simulink model "ModeInputHandle"  (R2018b)
settings: Solver=FixedStepDiscrete  StartTime=0.0  StopTime=10.0  FixedStep=0.01  RelTol=1e-3
undefined symbols (not defined in the file or in its folder): c, CmprtMdHMIReqExt2Tp1, CmprtMdHMIReqExtTp1, CmprtMdHMIReqTp1, d, e, EZESwReq1, f, g, IfVeSMSeStNumConfig, j, KeSMSuButtonLongPressedThrshldTm_Val, KeSMSuFoldType_Val, KeSMSwSeatSMSSeatMdTrigGapTimer_Val, KeSMSwSeatTrigWaitTimer_Val, KeSMSwSRSActiveValidTm_Val, LckUlckActvtFunc1, LstLckFunc1, LugSelectSw1, MdReqTp1, PowerMode1, SeatOccupiedSts1, SRSMode1, StPassCmprtMdCtrl_Md10_VCUConfig_Val, StPassCmprtMdCtrl_Md11_VCUConfig_Val, StPassCmprtMdCtrl_Md12_VCUConfig_Val, StPassCmprtMdCtrl_Md13_VCUConfig_Val, StPassCmprtMdCtrl_Md1_VCUConfig_Val, StPassCmprtMdCtrl_Md27_VCUConfig_Val, StPassCmprtMdCtrl_Md28_VCUConfig_Val, StPassCmprtMdCtrl_Md29_VCUConfig_Val, StPassCmprtMdCtrl_Md2_VCUConfig_Val, StPassCmprtMdCtrl_Md30_VCUConfig_Val, StPassCmprtMdCtrl_Md31_VCUConfig_Val, StPassCmprtMdCtrl_Md32_VCUConfig_Val, StPassCmprtMdCtrl_Md3_VCUConfig_Val, StPassCmprtMdCtrl_Md53_VCUConfig_Val, StPassCmprtMdCtrl_Md56_VCUConfig_Val, StPassCmprtMdCtrl_Md57_VCUConfig_Val, StPassCmprtMdCtrl_Md58_VCUConfig_Val, StPassCmprtMdCtrl_Md61_VCUConfig_Val, StPassCmprtMdCtrl_Md62_VCUConfig_Val, StPassCmprtMdCtrl_Md8_VCUConfig_Val, StPassCmprtMdCtrl_Md9_VCUConfig_Val, StSrv_StMd10_Config_Val, StSrv_StMd11_Config_Val, StSrv_StMd12_Config_Val, StSrv_StMd13_Config_Val, StSrv_StMd1_Config_Val, StSrv_StMd27_Config_Val, StSrv_StMd28_Config_Val, StSrv_StMd29_Config_Val, StSrv_StMd2_Config_Val, StSrv_StMd30_Config_Val, StSrv_StMd31_Config_Val, StSrv_StMd32_Config_Val, StSrv_StMd3_Config_Val, StSrv_StMd8_Config_Val, StSrv_StMd9_Config_Val, VehMovState1
libraries: MSMLib x91
(part 6 of 9)

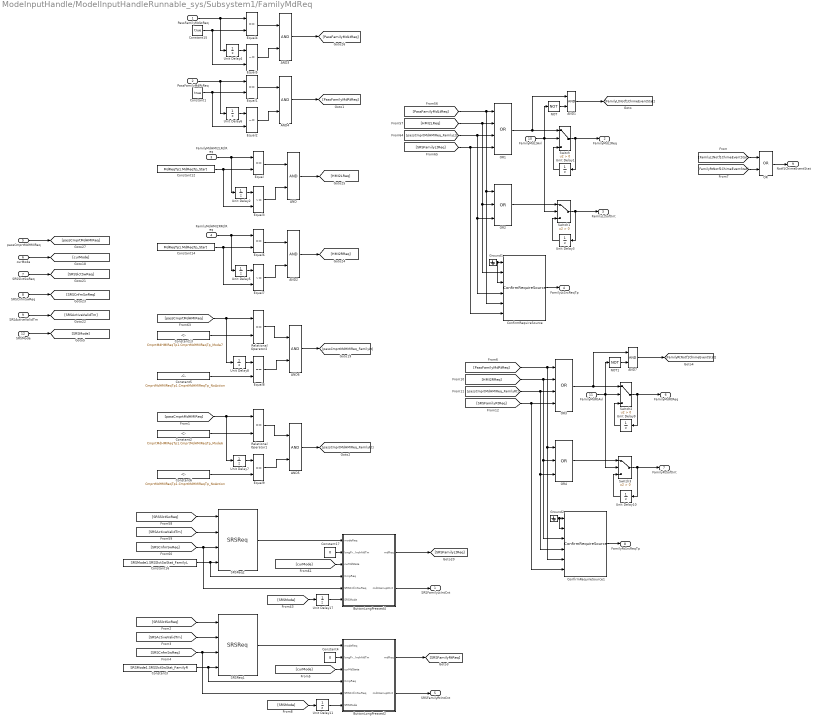
== system ModeInputHandle/ModelInputHandleRunnable_sys/Subsystem1/FamilyMdReq ==
  PassFamilyMdLtReq : Inport
  PassFamilyMdRtReq : Inport  Port=2
  FamilyMdHMI2LRclReq : Inport  Port=3
  FamilyMdHMI2RRclReq : Inport  Port=4
  passCmprtMdHMIReq : Inport  Port=5
  curMode : Inport  Port=6
  SRSSlctSwReq : Inport  Port=7
  SRSCnfmSwReq : Inport  Port=8
  SRSActiveValidTm : Inport  Port=9
  FamilyMdLtAvl : Inport  Port=10
  FamilyMdRtAvl : Inport  Port=11
  SRSMode : Inport  Port=12
  AND{,1..7} (8 alike) : Logic  AllPortsSameDT=off  OutDataTypeStr=boolean
  ButtonLongPressed2 : Subsystem  AncestorBlock=MSMLib/ButtonLongPressed
  ButtonLongPressed4 : Subsystem  AncestorBlock=MSMLib/ButtonLongPressed
  ConfirmRequireSource : MSMLib/ConfirmRequireSource  SystemSampleTime=-1
  ConfirmRequireSource1 : MSMLib/ConfirmRequireSource  SystemSampleTime=-1
  Constant1 : Constant  Value=true  OutDataTypeStr=boolean
  Constant12 : Constant  Value=MdReqTp1.MdReqTp_Start
  Constant13 : Constant  Value=CmprtMdHMIReqTp1.CmprtMdHMIReqTp_Mode7  OutDataTypeStr=Enum:CmprtMdHMIReqTp1
  Constant14 : Constant  Value=MdReqTp1.MdReqTp_Start
  Constant15 : Constant  Value=true  OutDataTypeStr=boolean
  Constant16 : Constant  Value=SRSMode1.SRSSlctSwStat_FamilyL  OutDataTypeStr=Enum:SRSMode1
  Constant17 : Constant  Value=0  OutDataTypeStr=uint8
  Constant2 : Constant  Value=CmprtMdHMIReqTp1.CmprtMdHMIReqTp_Mode6  OutDataTypeStr=Enum:CmprtMdHMIReqTp1
  Constant3 : Constant  Value=SRSMode1.SRSSlctSwStat_FamilyR  OutDataTypeStr=Enum:SRSMode1
  Constant4 : Constant  Value=0  OutDataTypeStr=uint8
  Constant5 : Constant  Value=CmprtMdHMIReqTp1.CmprtMdHMIReqTp_NoAction  OutDataTypeStr=Enum:CmprtMdHMIReqTp1
  Constant6 : Constant  Value=CmprtMdHMIReqTp1.CmprtMdHMIReqTp_NoAction  OutDataTypeStr=Enum:CmprtMdHMIReqTp1
  Equal{,1,4,6,8..9} (6 alike) : RelationalOperator  Operator===  OutDataTypeStr=boolean  RndMeth=Simplest
  Equal{2..3,5,7} (4 alike) : RelationalOperator  Operator=~=  OutDataTypeStr=boolean  RndMeth=Simplest
  Ground1 : Ground
  Ground2 : Ground
  NOT : Logic  Operator=NOT  AllPortsSameDT=off  OutDataTypeStr=boolean
  NOT1 : Logic  Operator=NOT  AllPortsSameDT=off  OutDataTypeStr=boolean
  OR : Logic  Operator=OR  AllPortsSameDT=off  OutDataTypeStr=boolean
  OR1 : Logic  Operator=OR  Inputs=4  AllPortsSameDT=off  OutDataTypeStr=boolean
  OR2 : Logic  Operator=OR  Inputs=3  AllPortsSameDT=off  OutDataTypeStr=boolean
  OR3 : Logic  Operator=OR  Inputs=4  AllPortsSameDT=off  OutDataTypeStr=boolean
  OR4 : Logic  Operator=OR  Inputs=3  AllPortsSameDT=off  OutDataTypeStr=boolean
  Relational Operator1 : RelationalOperator  Operator===  OutDataTypeStr=boolean  RndMeth=Simplest
  Relational Operator2 : RelationalOperator  Operator===  OutDataTypeStr=boolean  RndMeth=Simplest
  SRSReq1 : MSMLib/SRSReq  SystemSampleTime=-1
  SRSReq2 : MSMLib/SRSReq  SystemSampleTime=-1
  Switch{,1..3} (4 alike) : Switch  Criteria=u2 > Threshold
  Unit Delay{1,3..4,6,9..10} (6 alike) : UnitDelay  SampleTime=-1
  Unit Delay11 : UnitDelay  InitialCondition=d  SampleTime=-1
  Unit Delay17 : UnitDelay  InitialCondition=d  SampleTime=-1
  Unit Delay2 : UnitDelay  InitialCondition=e  SampleTime=-1
  Unit Delay5 : UnitDelay  InitialCondition=e  SampleTime=-1
  Unit Delay7 : UnitDelay  InitialCondition=c  SampleTime=-1
  Unit Delay8 : UnitDelay  InitialCondition=c  SampleTime=-1
  SRSFamilyLtIntCnt : Outport
  FamilyMdLtReq : Outport  Port=2
  FamilyLtSoftInt : Outport  Port=3
  FamilyLtSrcReqTp : Outport  Port=4
  SRSFamilyRtIntCnt : Outport  Port=5
  FamilyMdRtReq : Outport  Port=6
  FamilyRtSoftInt : Outport  Port=7
  FamilyRtSrcReqTp : Outport  Port=8
  Notf1ChimeEventStat : Outport  Port=9
  wires:
  FamilyMdLtAvl/1 -> Switch1/2, NOT/1, Switch/2
  [SRSActiveValidTm] -> SRSReq2/2
  Unit Delay2/1 -> Equal3/1
  FamilyMdHMI2LRclReq/1 -> Unit Delay2/1, Equal/1
  Constant14/1 -> Equal7/2, Equal6/2
  Equal5/1 -> AND3/2
  Constant16/1 -> ButtonLongPressed4/4(CmpReq), SRSReq2/4
  Equal6/1 -> AND2/1
  Equal/1 -> AND/1
  AND3/1 -> [PassFamilyMdLtReq]
  PassFamilyMdLtReq/1 -> Unit Delay4/1, Equal4/1
  [SRSCnfmSwReq] -> ButtonLongPressed4/5(SRSCnfmSwReq), SRSReq2/3
  Constant17/1 -> ButtonLongPressed4/2(longPressThrshhldTm)
  [PassFamilyMdLtReq] -> ConfirmRequireSource/5, OR2/1, OR1/1
  Equal3/1 -> AND/2
  SRSSlctSwReq/1 -> [SRSSlctSwReq]
  OR1/1 -> AND1/1, Switch/1
  FamilyMdHMI2RRclReq/1 -> Unit Delay5/1, Equal6/1
  Constant13/1 -> Relational Operator2/2
  [curMode] -> ButtonLongPressed4/3(curMdState)
  Equal4/1 -> AND3/1
  Constant12/1 -> Equal3/2, Equal/2
  curMode/1 -> [curMode]
  [passCmprtMdHMIReq] -> Unit Delay8/1, Relational Operator2/1
  AND1/1 -> [FamilyLtNotf1ChimeEventStat]
  SRSActiveValidTm/1 -> [SRSActiveValidTm]
  OR2/1 -> Switch1/1
  Equal7/1 -> AND2/2
  Switch/1 -> FamilyMdLtReq/1, Unit Delay1/1
  Constant15/1 -> Equal4/2, Equal5/2
  Unit Delay5/1 -> Equal7/1
  ButtonLongPressed4/1(mdReq) -> [SRSFamilyLtReq]
  Unit Delay1/1 -> Switch/3
  AND6/1 -> [passCmprtMdHMIReq_FamilyLt]
  ConfirmRequireSource/1 -> FamilyLtSrcReqTp/1
  SRSCnfmSwReq/1 -> [SRSCnfmSwReq]
  Switch1/1 -> FamilyLtSoftInt/1, Unit Delay3/1
  Ground1/1 -> ConfirmRequireSource/3, ConfirmRequireSource/1
  Unit Delay4/1 -> Equal5/1
  NOT/1 -> AND1/2
  ButtonLongPressed4/2(mdInterruptCnt) -> SRSFamilyLtIntCnt/1
  AND2/1 -> [HMI2RReq]
  Unit Delay8/1 -> Equal8/1
  [SRSSlctSwReq] -> SRSReq2/1
  Equal8/1 -> AND6/2
  AND/1 -> [HMI2LReq]
  SRSReq2/1 -> ButtonLongPressed4/1(modeReq)
  passCmprtMdHMIReq/1 -> [passCmprtMdHMIReq]
  Unit Delay3/1 -> Switch1/3
  Relational Operator2/1 -> AND6/1
  Unit Delay6/1 -> Equal2/1
  Equal1/1 -> AND4/1
  Equal2/1 -> AND4/2
  PassFamilyMdRtReq/1 -> Unit Delay6/1, Equal1/1
  Constant1/1 -> Equal1/2, Equal2/2
  AND4/1 -> [PassFamilyMdRtReq]
  [passCmprtMdHMIReq] -> Unit Delay7/1, Relational Operator1/1
  Relational Operator1/1 -> AND5/1
  Equal9/1 -> AND5/2
  Constant2/1 -> Relational Operator1/2
  Unit Delay7/1 -> Equal9/1
  AND5/1 -> [passCmprtMdHMIReq_FamilyRt]
  SRSReq1/1 -> ButtonLongPressed2/1(modeReq)
  [SRSSlctSwReq] -> SRSReq1/1
  [curMode] -> ButtonLongPressed2/3(curMdState)
  Constant4/1 -> ButtonLongPressed2/2(longPressThrshhldTm)
  [SRSActiveValidTm] -> SRSReq1/2
  Constant3/1 -> ButtonLongPressed2/4(CmpReq), SRSReq1/4
  ButtonLongPressed2/1(mdReq) -> [SRSFamilyRtReq]
  [SRSCnfmSwReq] -> ButtonLongPressed2/5(SRSCnfmSwReq), SRSReq1/3
  ButtonLongPressed2/2(mdInterruptCnt) -> SRSFamilyRtIntCnt/1
  [HMI2LReq] -> ConfirmRequireSource/2, OR2/2, OR1/2
  [passCmprtMdHMIReq_FamilyLt] -> ConfirmRequireSource/4, OR2/3, OR1/3
  [SRSFamilyLtReq] -> ConfirmRequireSource/6, OR1/4
  Switch3/1 -> FamilyRtSoftInt/1, Unit Delay10/1
  Unit Delay10/1 -> Switch3/3
  NOT1/1 -> AND7/2
  OR3/1 -> AND7/1, Switch2/1
  [PassFamilyMdRtReq] -> ConfirmRequireSource1/5, OR4/1, OR3/1
  [passCmprtMdHMIReq_FamilyRt] -> ConfirmRequireSource1/4, OR4/3, OR3/3
  Ground2/1 -> ConfirmRequireSource1/2, ConfirmRequireSource1/1
  ConfirmRequireSource1/1 -> FamilyRtSrcReqTp/1
  [SRSFamilyRtReq] -> ConfirmRequireSource1/6, OR3/4
  Switch2/1 -> FamilyMdRtReq/1, Unit Delay9/1
  OR4/1 -> Switch3/1
  FamilyMdRtAvl/1 -> Switch3/2, NOT1/1, Switch2/2
  Unit Delay9/1 -> Switch2/3
  AND7/1 -> [FamilyRtNotf1ChimeEventStat]
  [HMI2RReq] -> ConfirmRequireSource1/3, OR4/2, OR3/2
  [FamilyLtNotf1ChimeEventStat] -> OR/1
  [FamilyRtNotf1ChimeEventStat] -> OR/2
  OR/1 -> Notf1ChimeEventStat/1
  Unit Delay17/1 -> ButtonLongPressed4/6(SRSMode)
  [SRSMode] -> Unit Delay17/1
  Unit Delay11/1 -> ButtonLongPressed2/6(SRSMode)
  [SRSMode] -> Unit Delay11/1
  SRSMode/1 -> [SRSMode]
  Constant5/1 -> Equal8/2
  Constant6/1 -> Equal9/2

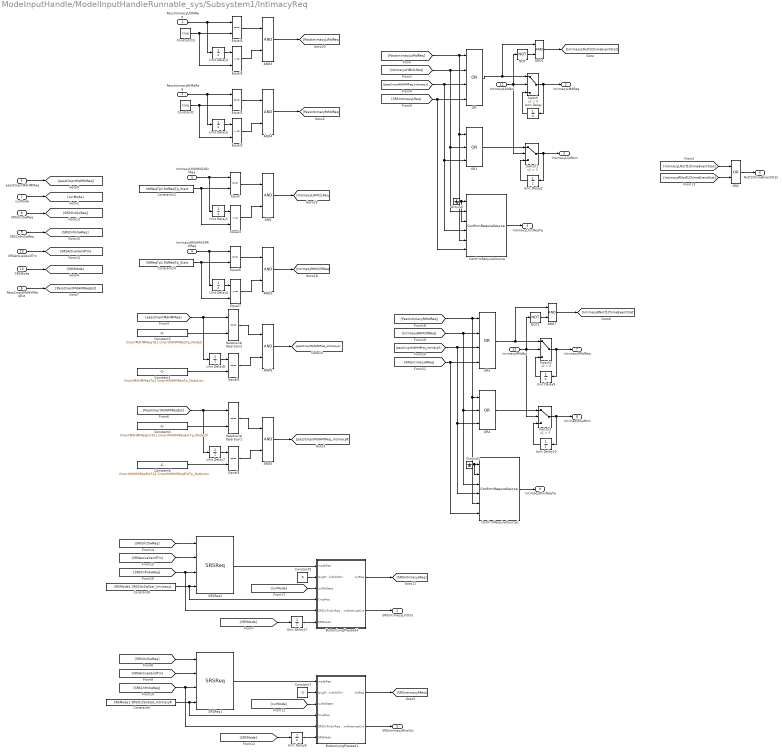
== system ModeInputHandle/ModelInputHandleRunnable_sys/Subsystem1/IntimacyReq ==
  PassIntimacyLtMdReq : Inport
  PassIntimacyRtMdReq : Inport  Port=2
  IntimacyLMdHMI2LRclReq : Inport  Port=3
  IntimacyRMdHMI2RRclReq : Inport  Port=4
  passCmprtMdHMIReq : Inport  Port=5
  PassCmprtMdHMIReqExt : Inport  Port=6
  curMode : Inport  Port=7
  SRSSlctSwReq : Inport  Port=8
  SRSCnfmSwReq : Inport  Port=9
  SRSActiveValidTm : Inport  Port=10
  IntimacyLMdAvl : Inport  Port=11
  IntimacyRMdAvl : Inport  Port=12
  SRSMode : Inport  Port=13
  AND{,1..7} (8 alike) : Logic  AllPortsSameDT=off  OutDataTypeStr=boolean
  ButtonLongPressed1 : Subsystem  AncestorBlock=MSMLib/ButtonLongPressed
  ButtonLongPressed4 : Subsystem  AncestorBlock=MSMLib/ButtonLongPressed
  ConfirmRequireSource : MSMLib/ConfirmRequireSource  SystemSampleTime=-1
  ConfirmRequireSource1 : MSMLib/ConfirmRequireSource  SystemSampleTime=-1
  Constant1 : Constant  Value=CmprtMdHMIReqTp1.CmprtMdHMIReqTp_NoAction  OutDataTypeStr=Enum:CmprtMdHMIReqTp1
  Constant12 : Constant  Value=MdReqTp1.MdReqTp_Start
  Constant14 : Constant  Value=MdReqTp1.MdReqTp_Start
  Constant15 : Constant  Value=true  OutDataTypeStr=boolean
  Constant2 : Constant  Value=true  OutDataTypeStr=boolean
  Constant3 : Constant  Value=CmprtMdHMIReqTp1.CmprtMdHMIReqTp_Mode5  OutDataTypeStr=Enum:CmprtMdHMIReqTp1
  Constant4 : Constant  Value=CmprtMdHMIReqExtTp1.CmprtMdHMIReqExtTp_Mode20  OutDataTypeStr=Enum:CmprtMdHMIReqExtTp1
  Constant5 : Constant  Value=SRSMode1.SRSSlctSwStat_IntimacyR  OutDataTypeStr=Enum:SRSMode1
  Constant6 : Constant  Value=CmprtMdHMIReqExtTp1.CmprtMdHMIReqExtTp_NoAction  OutDataTypeStr=Enum:CmprtMdHMIReqExtTp1
  Constant7 : Constant  Value=0  OutDataTypeStr=uint8
  Constant8 : Constant  Value=SRSMode1.SRSSlctSwStat_IntimacyL  OutDataTypeStr=Enum:SRSMode1
  Constant9 : Constant  Value=0  OutDataTypeStr=uint8
  Equal{,1,4,6,8..9} (6 alike) : RelationalOperator  Operator===  OutDataTypeStr=boolean  RndMeth=Simplest
  Equal{2..3,5,7} (4 alike) : RelationalOperator  Operator=~=  OutDataTypeStr=boolean  RndMeth=Simplest
  Ground : Ground
  Ground1 : Ground
  NOT : Logic  Operator=NOT  AllPortsSameDT=off  OutDataTypeStr=boolean
  NOT1 : Logic  Operator=NOT  AllPortsSameDT=off  OutDataTypeStr=boolean
  OR : Logic  Operator=OR  Inputs=4  AllPortsSameDT=off  OutDataTypeStr=boolean
  OR1 : Logic  Operator=OR  Inputs=3  AllPortsSameDT=off  OutDataTypeStr=boolean
  OR2 : Logic  Operator=OR  AllPortsSameDT=off  OutDataTypeStr=boolean
  OR3 : Logic  Operator=OR  Inputs=4  AllPortsSameDT=off  OutDataTypeStr=boolean
  OR4 : Logic  Operator=OR  Inputs=3  AllPortsSameDT=off  OutDataTypeStr=boolean
  Relational Operator1 : RelationalOperator  Operator===  OutDataTypeStr=boolean  RndMeth=Simplest
  Relational Operator2 : RelationalOperator  Operator===  OutDataTypeStr=boolean  RndMeth=Simplest
  SRSReq1 : MSMLib/SRSReq  SystemSampleTime=-1
  SRSReq2 : MSMLib/SRSReq  SystemSampleTime=-1
  Switch{,1..3} (4 alike) : Switch  Criteria=u2 > Threshold
  Unit Delay{,2..3,5,9..10} (6 alike) : UnitDelay  SampleTime=-1
  Unit Delay1 : UnitDelay  InitialCondition=e  SampleTime=-1
  Unit Delay17 : UnitDelay  InitialCondition=d  SampleTime=-1
  Unit Delay4 : UnitDelay  InitialCondition=e  SampleTime=-1
  Unit Delay6 : UnitDelay  InitialCondition=d  SampleTime=-1
  Unit Delay7 : UnitDelay  InitialCondition=g  SampleTime=-1
  Unit Delay8 : UnitDelay  InitialCondition=c  SampleTime=-1
  SRSIntimacyLIntCnt : Outport
  IntimacyLMdReq : Outport  Port=2
  IntimacyLSoftInt : Outport  Port=3
  IntimacyLSrcReqTp : Outport  Port=4
  SRSIntimacyRIntCnt : Outport  Port=5
  "Notf1ChimeEventStat " : Outport  Port=6
  IntimacyRMdReq : Outport  Port=7
  IntimacyRSoftInt : Outport  Port=8
  IntimacyRSrcReqTp : Outport  Port=9
  wires:
  AND2/1 -> [IntimacyRHMI2RReq]
  Constant12/1 -> Equal3/2, Equal/2
  Unit Delay1/1 -> Equal3/1
  PassIntimacyLtMdReq/1 -> Unit Delay3/1, Equal4/1
  Equal/1 -> AND/1
  IntimacyLMdHMI2LRclReq/1 -> Unit Delay1/1, Equal/1
  AND/1 -> [IntimacyLHMI2LReq]
  Unit Delay3/1 -> Equal5/1
  AND3/1 -> [PassIntimacyLtMdReq]
  Equal5/1 -> AND3/2
  Constant14/1 -> Equal7/2, Equal6/2
  Equal7/1 -> AND2/2
  IntimacyRMdHMI2RRclReq/1 -> Unit Delay4/1, Equal6/1
  Equal4/1 -> AND3/1
  Equal3/1 -> AND/2
  Constant15/1 -> Equal4/2, Equal5/2
  Unit Delay4/1 -> Equal7/1
  Equal6/1 -> AND2/1
  Constant3/1 -> Relational Operator2/2
  Relational Operator2/1 -> AND6/1
  Unit Delay8/1 -> Equal8/1
  Equal8/1 -> AND6/2
  [passCmprtMdHMIReq] -> Unit Delay8/1, Relational Operator2/1
  AND6/1 -> [passCmprtMdHMIReq_IntimacyL]
  passCmprtMdHMIReq/1 -> [passCmprtMdHMIReq]
  [SRSCnfmSwReq] -> ButtonLongPressed4/5(SRSCnfmSwReq), SRSReq2/3
  SRSReq2/1 -> ButtonLongPressed4/1(modeReq)
  Constant9/1 -> ButtonLongPressed4/2(longPressThrshhldTm)
  [curMode] -> ButtonLongPressed4/3(curMdState)
  Constant8/1 -> ButtonLongPressed4/4(CmpReq), SRSReq2/4
  [SRSSlctSwReq] -> SRSReq2/1
  [SRSActiveValidTm] -> SRSReq2/2
  ButtonLongPressed4/2(mdInterruptCnt) -> SRSIntimacyLIntCnt/1
  ButtonLongPressed4/1(mdReq) -> [SRSIntimacyLReq]
  SRSCnfmSwReq/1 -> [SRSCnfmSwReq]
  SRSSlctSwReq/1 -> [SRSSlctSwReq]
  curMode/1 -> [curMode]
  SRSActiveValidTm/1 -> [SRSActiveValidTm]
  [SRSIntimacyLReq] -> OR/4, ConfirmRequireSource/6
  [IntimacyLHMI2LReq] -> OR/2, OR1/2, ConfirmRequireSource/2
  [PassIntimacyLtMdReq] -> OR/1, ConfirmRequireSource/5, OR1/1
  OR/1 -> AND1/1, Switch/1
  IntimacyLMdAvl/1 -> Switch1/2, NOT/1, Switch/2
  Switch/1 -> IntimacyLMdReq/1, Unit Delay/1
  Unit Delay/1 -> Switch/3
  NOT/1 -> AND1/2
  OR1/1 -> Switch1/1
  Switch1/1 -> IntimacyLSoftInt/1, Unit Delay2/1
  Unit Delay2/1 -> Switch1/3
  [passCmprtMdHMIReq_IntimacyL] -> OR/3, OR1/3, ConfirmRequireSource/4
  Ground/1 -> ConfirmRequireSource/3, ConfirmRequireSource/1
  ConfirmRequireSource/1 -> IntimacyLSrcReqTp/1
  Unit Delay17/1 -> ButtonLongPressed4/6(SRSMode)
  Constant1/1 -> Equal8/2
  Equal1/1 -> AND4/1
  Constant2/1 -> Equal1/2, Equal2/2
  PassIntimacyRtMdReq/1 -> Unit Delay5/1, Equal1/1
  Unit Delay5/1 -> Equal2/1
  Equal2/1 -> AND4/2
  AND4/1 -> [PassIntimacyRtMdReq]
  [PassCmprtMdHMIReqExt] -> Unit Delay7/1, Relational Operator1/1
  AND5/1 -> [passCmprtMdHMIReq_IntimacyR]
  Equal9/1 -> AND5/2
  Unit Delay7/1 -> Equal9/1
  Constant6/1 -> Equal9/2
  Relational Operator1/1 -> AND5/1
  Constant4/1 -> Relational Operator1/2
  SRSMode/1 -> [SRSMode]
  [SRSMode] -> Unit Delay17/1
  [SRSMode] -> Unit Delay6/1
  [SRSActiveValidTm] -> SRSReq1/2
  Unit Delay6/1 -> ButtonLongPressed1/6(SRSMode)
  Constant7/1 -> ButtonLongPressed1/2(longPressThrshhldTm)
  ButtonLongPressed1/1(mdReq) -> [SRSIntimacyRReq]
  SRSReq1/1 -> ButtonLongPressed1/1(modeReq)
  [SRSSlctSwReq] -> SRSReq1/1
  Constant5/1 -> ButtonLongPressed1/4(CmpReq), SRSReq1/4
  ButtonLongPressed1/2(mdInterruptCnt) -> SRSIntimacyRIntCnt/1
  [curMode] -> ButtonLongPressed1/3(curMdState)
  [SRSCnfmSwReq] -> ButtonLongPressed1/5(SRSCnfmSwReq), SRSReq1/3
  [IntimacyRNotf1ChimeEventStat] -> OR2/2
  OR2/1 -> "Notf1ChimeEventStat "/1
  [IntimacyLNotf1ChimeEventStat] -> OR2/1
  [passCmprtMdHMIReq_IntimacyR] -> OR3/3, OR4/3, ConfirmRequireSource1/4
  OR3/1 -> AND7/1, Switch2/1
  Unit Delay10/1 -> Switch3/3
  AND7/1 -> [IntimacyRNotf1ChimeEventStat]
  OR4/1 -> Switch3/1
  Unit Delay9/1 -> Switch2/3
  IntimacyRMdAvl/1 -> NOT1/1, Switch3/2, Switch2/2
  ConfirmRequireSource1/1 -> IntimacyRSrcReqTp/1
  Ground1/1 -> ConfirmRequireSource1/2, ConfirmRequireSource1/1
  [PassIntimacyRtMdReq] -> OR3/1, ConfirmRequireSource1/5, OR4/1
  Switch2/1 -> IntimacyRMdReq/1, Unit Delay9/1
  NOT1/1 -> AND7/2
  [IntimacyRHMI2RReq] -> OR3/2, ConfirmRequireSource1/3, OR4/2
  [SRSIntimacyRReq] -> OR3/4, ConfirmRequireSource1/6
  Switch3/1 -> IntimacyRSoftInt/1, Unit Delay10/1
  AND1/1 -> [IntimacyLNotf1ChimeEventStat]
  PassCmprtMdHMIReqExt/1 -> [PassCmprtMdHMIReqExt]

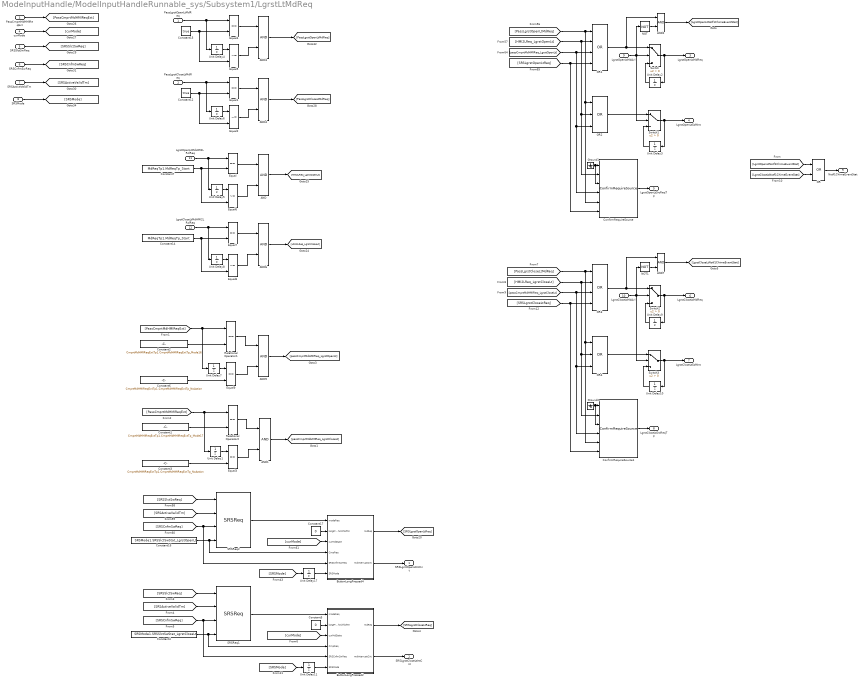
== system ModeInputHandle/ModelInputHandleRunnable_sys/Subsystem1/LgrstLtMdReq ==
  PassLgrstOpenLtMdReq : Inport
  PassLgrstCloseLtMdReq : Inport  Port=2
  PassCmprtMdHMIReqExt : Inport  Port=3
  curMode : Inport  Port=4
  SRSSlctSwReq : Inport  Port=5
  SRSCnfmSwReq : Inport  Port=6
  SRSActiveValidTm : Inport  Port=7
  SRSMode : Inport  Port=8
  LgrstOpenLtMdAvl : Inport  Port=9
  LgrstCloseLtMdAvl : Inport  Port=10
  LgrstOpenLtMdHMI2LRclReq : Inport  Port=11
  LgrstCloseLtMdHMI2LRclReq : Inport  Port=12
  AND{,1..7} (8 alike) : Logic  AllPortsSameDT=off  OutDataTypeStr=boolean
  ButtonLongPressed2 : Subsystem  AncestorBlock=MSMLib/ButtonLongPressed
  ButtonLongPressed4 : Subsystem  AncestorBlock=MSMLib/ButtonLongPressed
  ConfirmRequireSource : MSMLib/ConfirmRequireSource  SystemSampleTime=-1
  ConfirmRequireSource1 : MSMLib/ConfirmRequireSource  SystemSampleTime=-1
  Constant1 : Constant  Value=CmprtMdHMIReqExtTp1.CmprtMdHMIReqExtTp_Mode17  OutDataTypeStr=Enum:CmprtMdHMIReqExtTp1
  Constant12 : Constant  Value=true  OutDataTypeStr=boolean
  Constant14 : Constant  Value=MdReqTp1.MdReqTp_Start
  Constant15 : Constant  Value=true  OutDataTypeStr=boolean
  Constant16 : Constant  Value=SRSMode1.SRSSlctSwStat_LgrstOpenLt  OutDataTypeStr=Enum:SRSMode1
  Constant17 : Constant  Value=0  OutDataTypeStr=uint8
  Constant2 : Constant  Value=CmprtMdHMIReqExtTp1.CmprtMdHMIReqExtTp_Mode16  OutDataTypeStr=Enum:CmprtMdHMIReqExtTp1
  Constant3 : Constant  Value=CmprtMdHMIReqExtTp1.CmprtMdHMIReqExtTp_NoAction  OutDataTypeStr=Enum:CmprtMdHMIReqExtTp1
  Constant4 : Constant  Value=SRSMode1.SRSSlctSwStat_LgrstCloseLt  OutDataTypeStr=Enum:SRSMode1
  Constant5 : Constant  Value=0  OutDataTypeStr=uint8
  Constant6 : Constant  Value=CmprtMdHMIReqExtTp1.CmprtMdHMIReqExtTp_NoAction  OutDataTypeStr=Enum:CmprtMdHMIReqExtTp1
  Constant7 : Constant  Value=MdReqTp1.MdReqTp_Start
  Equal{,1,3..4,7,9} (6 alike) : RelationalOperator  Operator===  OutDataTypeStr=boolean  RndMeth=Simplest
  Equal{2,5..6,8} (4 alike) : RelationalOperator  Operator=~=  OutDataTypeStr=boolean  RndMeth=Simplest
  Ground1 : Ground
  Ground2 : Ground
  NOT : Logic  Operator=NOT  AllPortsSameDT=off  OutDataTypeStr=boolean
  NOT1 : Logic  Operator=NOT  AllPortsSameDT=off  OutDataTypeStr=boolean
  OR : Logic  Operator=OR  AllPortsSameDT=off  OutDataTypeStr=boolean
  OR1 : Logic  Operator=OR  Inputs=4  AllPortsSameDT=off  OutDataTypeStr=boolean
  OR2 : Logic  Operator=OR  Inputs=3  AllPortsSameDT=off  OutDataTypeStr=boolean
  OR3 : Logic  Operator=OR  Inputs=4  AllPortsSameDT=off  OutDataTypeStr=boolean
  OR4 : Logic  Operator=OR  Inputs=3  AllPortsSameDT=off  OutDataTypeStr=boolean
  Relational Operator1 : RelationalOperator  Operator===  OutDataTypeStr=boolean  RndMeth=Simplest
  Relational Operator2 : RelationalOperator  Operator===  OutDataTypeStr=boolean  RndMeth=Simplest
  SRSReq1 : MSMLib/SRSReq  SystemSampleTime=-1
  SRSReq2 : MSMLib/SRSReq  SystemSampleTime=-1
  Switch{,1..3} (4 alike) : Switch  Criteria=u2 > Threshold
  Unit Delay1 : UnitDelay  InitialCondition=g  SampleTime=-1
  Unit Delay{2..4,6,9..10} (6 alike) : UnitDelay  SampleTime=-1
  Unit Delay11 : UnitDelay  InitialCondition=d  SampleTime=-1
  Unit Delay17 : UnitDelay  InitialCondition=d  SampleTime=-1
  Unit Delay5 : UnitDelay  InitialCondition=e  SampleTime=-1
  Unit Delay7 : UnitDelay  InitialCondition=g  SampleTime=-1
  Unit Delay8 : UnitDelay  InitialCondition=e  SampleTime=-1
  SRSLgrstOpenLtIntCnt : Outport
  SRSLgrstCloseLtIntCnt : Outport  Port=2
  LgrstOpenLtMdReq : Outport  Port=3
  LgrstOpenLtSoftInt : Outport  Port=4
  LgrstOpenLtSrcReqTp : Outport  Port=5
  LgrstCloseLtMdReq : Outport  Port=6
  LgrstCloseLtSoftInt : Outport  Port=7
  LgrstCloseLtSrcReqTp : Outport  Port=8
  Notf1ChimeEventStat : Outport  Port=9
  wires:
  Constant12/1 -> Equal1/2, Equal2/2
  Equal2/1 -> AND4/2
  Equal4/1 -> AND3/1
  SRSActiveValidTm/1 -> [SRSActiveValidTm]
  curMode/1 -> [curMode]
  Equal1/1 -> AND4/1
  Constant15/1 -> Equal4/2, Equal5/2
  Unit Delay4/1 -> Equal5/1
  SRSSlctSwReq/1 -> [SRSSlctSwReq]
  PassLgrstOpenLtMdReq/1 -> Unit Delay4/1, Equal4/1
  SRSMode/1 -> [SRSMode]
  AND4/1 -> [PassLgrstCloseLtMdReq]
  AND3/1 -> [PassLgrstOpenLtMdReq]
  PassCmprtMdHMIReqExt/1 -> [PassCmprtMdHMIReqExt]
  Equal5/1 -> AND3/2
  PassLgrstCloseLtMdReq/1 -> Unit Delay6/1, Equal1/1
  Unit Delay6/1 -> Equal2/1
  SRSCnfmSwReq/1 -> [SRSCnfmSwReq]
  Relational Operator1/1 -> AND5/1
  Constant2/1 -> Relational Operator1/2
  Constant6/1 -> Equal9/2
  Unit Delay7/1 -> Equal9/1
  AND5/1 -> [passCmprtMdHMIReq_LgrstOpenLt]
  [PassCmprtMdHMIReqExt] -> Unit Delay7/1, Relational Operator1/1
  Equal9/1 -> AND5/2
  [PassCmprtMdHMIReqExt] -> Unit Delay1/1, Relational Operator2/1
  Equal3/1 -> AND1/2
  Constant3/1 -> Equal3/2
  Unit Delay1/1 -> Equal3/1
  AND1/1 -> [passCmprtMdHMIReq_LgrstCloseLt]
  Constant1/1 -> Relational Operator2/2
  Relational Operator2/1 -> AND1/1
  ButtonLongPressed2/2(mdInterruptCnt) -> SRSLgrstCloseLtIntCnt/1
  [SRSMode] -> Unit Delay17/1
  Unit Delay17/1 -> ButtonLongPressed4/6(SRSMode)
  Constant16/1 -> ButtonLongPressed4/4(CmpReq), SRSReq2/4
  [SRSActiveValidTm] -> SRSReq2/2
  ButtonLongPressed4/1(mdReq) -> [SRSLgrstOpenLtReq]
  [SRSCnfmSwReq] -> ButtonLongPressed4/5(SRSCnfmSwReq), SRSReq2/3
  [curMode] -> ButtonLongPressed2/3(curMdState)
  [SRSSlctSwReq] -> SRSReq2/1
  [curMode] -> ButtonLongPressed4/3(curMdState)
  Constant17/1 -> ButtonLongPressed4/2(longPressThrshhldTm)
  SRSReq2/1 -> ButtonLongPressed4/1(modeReq)
  [SRSCnfmSwReq] -> ButtonLongPressed2/5(SRSCnfmSwReq), SRSReq1/3
  Constant5/1 -> ButtonLongPressed2/2(longPressThrshhldTm)
  [SRSSlctSwReq] -> SRSReq1/1
  [SRSActiveValidTm] -> SRSReq1/2
  ButtonLongPressed2/1(mdReq) -> [SRSLgrstCloseLtReq]
  [SRSMode] -> Unit Delay11/1
  Constant4/1 -> ButtonLongPressed2/4(CmpReq), SRSReq1/4
  SRSReq1/1 -> ButtonLongPressed2/1(modeReq)
  ButtonLongPressed4/2(mdInterruptCnt) -> SRSLgrstOpenLtIntCnt/1
  Unit Delay11/1 -> ButtonLongPressed2/6(SRSMode)
  [passCmprtMdHMIReq_LgrstOpenLt] -> ConfirmRequireSource/4, OR2/3, OR1/3
  Ground2/1 -> ConfirmRequireSource1/3, ConfirmRequireSource1/1
  NOT/1 -> AND2/2
  Switch2/1 -> LgrstCloseLtMdReq/1, Unit Delay9/1
  [HMI2LReq_LgrstOpenLt] -> ConfirmRequireSource/2, OR2/2, OR1/2
  [PassLgrstCloseLtMdReq] -> ConfirmRequireSource1/5, OR4/1, OR3/1
  OR2/1 -> Switch1/1
  [LgrstOpenLtNotf1ChimeEventStat] -> OR/1
  OR/1 -> Notf1ChimeEventStat/1
  ConfirmRequireSource1/1 -> LgrstCloseLtSrcReqTp/1
  [HMI2LReq_LgrstCloseLt] -> ConfirmRequireSource1/2, OR4/2, OR3/2
  LgrstCloseLtMdAvl/1 -> Switch3/2, NOT1/1, Switch2/2
  OR3/1 -> AND7/1, Switch2/1
  OR4/1 -> Switch3/1
  OR1/1 -> AND2/1, Switch/1
  [PassLgrstOpenLtMdReq] -> ConfirmRequireSource/5, OR2/1, OR1/1
  Switch1/1 -> LgrstOpenLtSoftInt/1, Unit Delay3/1
  Switch3/1 -> LgrstCloseLtSoftInt/1, Unit Delay10/1
  LgrstOpenLtMdAvl/1 -> Switch1/2, NOT/1, Switch/2
  [SRSLgrstCloseLtReq] -> ConfirmRequireSource1/6, OR3/4
  Unit Delay10/1 -> Switch3/3
  Unit Delay9/1 -> Switch2/3
  Unit Delay2/1 -> Switch/3
  [LgrstCloseLtNotf1ChimeEventStat] -> OR/2
  AND2/1 -> [LgrstOpenLtNotf1ChimeEventStat]
  AND7/1 -> [LgrstCloseLtNotf1ChimeEventStat]
  [SRSLgrstOpenLtReq] -> ConfirmRequireSource/6, OR1/4
  Ground1/1 -> ConfirmRequireSource/3, ConfirmRequireSource/1
  Switch/1 -> LgrstOpenLtMdReq/1, Unit Delay2/1
  NOT1/1 -> AND7/2
  Unit Delay3/1 -> Switch1/3
  [passCmprtMdHMIReq_LgrstCloseLt] -> ConfirmRequireSource1/4, OR4/3, OR3/3
  ConfirmRequireSource/1 -> LgrstOpenLtSrcReqTp/1
  Constant14/1 -> Equal8/2, Equal7/2
  LgrstOpenLtMdHMI2LRclReq/1 -> Unit Delay5/1, Equal/1
  Unit Delay5/1 -> Equal6/1
  Equal6/1 -> AND/2
  AND6/1 -> [HMI2LReq_LgrstCloseLt]
  Unit Delay8/1 -> Equal8/1
  Equal8/1 -> AND6/2
  AND/1 -> [HMI2LReq_LgrstOpenLt]
  Equal7/1 -> AND6/1
  Equal/1 -> AND/1
  Constant7/1 -> Equal6/2, Equal/2
  LgrstCloseLtMdHMI2LRclReq/1 -> Unit Delay8/1, Equal7/1

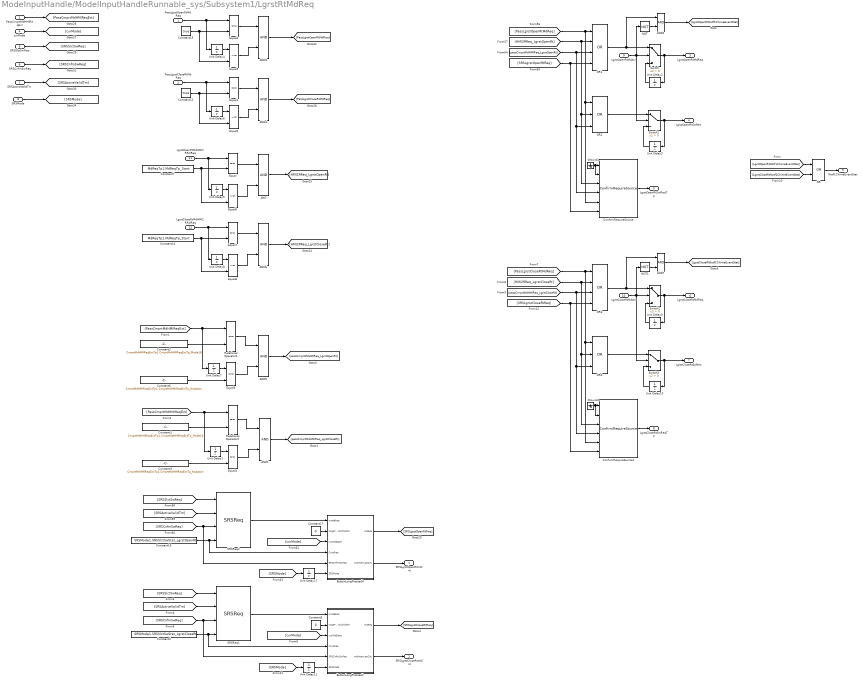
== system ModeInputHandle/ModelInputHandleRunnable_sys/Subsystem1/LgrstRtMdReq ==
  PassLgrstOpenRtMdReq : Inport
  PassLgrstCloseRtMdReq : Inport  Port=2
  PassCmprtMdHMIReqExt : Inport  Port=3
  curMode : Inport  Port=4
  SRSSlctSwReq : Inport  Port=5
  SRSCnfmSwReq : Inport  Port=6
  SRSActiveValidTm : Inport  Port=7
  SRSMode : Inport  Port=8
  LgrstOpenRtMdAvl : Inport  Port=9
  LgrstCloseRtMdAvl : Inport  Port=10
  LgrstOpenRtMdHMI2RRclReq : Inport  Port=11
  LgrstCloseRtMdHMI2RRclReq : Inport  Port=12
  AND{,1..7} (8 alike) : Logic  AllPortsSameDT=off  OutDataTypeStr=boolean
  ButtonLongPressed2 : Subsystem  AncestorBlock=MSMLib/ButtonLongPressed
  ButtonLongPressed4 : Subsystem  AncestorBlock=MSMLib/ButtonLongPressed
  ConfirmRequireSource : MSMLib/ConfirmRequireSource  SystemSampleTime=-1
  ConfirmRequireSource1 : MSMLib/ConfirmRequireSource  SystemSampleTime=-1
  Constant1 : Constant  Value=CmprtMdHMIReqExtTp1.CmprtMdHMIReqExtTp_Mode19  OutDataTypeStr=Enum:CmprtMdHMIReqExtTp1
  Constant12 : Constant  Value=true  OutDataTypeStr=boolean
  Constant14 : Constant  Value=MdReqTp1.MdReqTp_Start
  Constant15 : Constant  Value=true  OutDataTypeStr=boolean
  Constant16 : Constant  Value=SRSMode1.SRSSlctSwStat_LgrstOpenRt  OutDataTypeStr=Enum:SRSMode1
  Constant17 : Constant  Value=0  OutDataTypeStr=uint8
  Constant2 : Constant  Value=CmprtMdHMIReqExtTp1.CmprtMdHMIReqExtTp_Mode18  OutDataTypeStr=Enum:CmprtMdHMIReqExtTp1
  Constant3 : Constant  Value=CmprtMdHMIReqExtTp1.CmprtMdHMIReqExtTp_NoAction  OutDataTypeStr=Enum:CmprtMdHMIReqExtTp1
  Constant4 : Constant  Value=SRSMode1.SRSSlctSwStat_LgrstCloseRt  OutDataTypeStr=Enum:SRSMode1
  Constant5 : Constant  Value=0  OutDataTypeStr=uint8
  Constant6 : Constant  Value=CmprtMdHMIReqExtTp1.CmprtMdHMIReqExtTp_NoAction  OutDataTypeStr=Enum:CmprtMdHMIReqExtTp1
  Constant7 : Constant  Value=MdReqTp1.MdReqTp_Start
  Equal{,1,3..4,7,9} (6 alike) : RelationalOperator  Operator===  OutDataTypeStr=boolean  RndMeth=Simplest
  Equal{2,5..6,8} (4 alike) : RelationalOperator  Operator=~=  OutDataTypeStr=boolean  RndMeth=Simplest
  Ground1 : Ground
  Ground2 : Ground
  NOT : Logic  Operator=NOT  AllPortsSameDT=off  OutDataTypeStr=boolean
  NOT1 : Logic  Operator=NOT  AllPortsSameDT=off  OutDataTypeStr=boolean
  OR : Logic  Operator=OR  AllPortsSameDT=off  OutDataTypeStr=boolean
  OR1 : Logic  Operator=OR  Inputs=4  AllPortsSameDT=off  OutDataTypeStr=boolean
  OR2 : Logic  Operator=OR  Inputs=3  AllPortsSameDT=off  OutDataTypeStr=boolean
  OR3 : Logic  Operator=OR  Inputs=4  AllPortsSameDT=off  OutDataTypeStr=boolean
  OR4 : Logic  Operator=OR  Inputs=3  AllPortsSameDT=off  OutDataTypeStr=boolean
  Relational Operator1 : RelationalOperator  Operator===  OutDataTypeStr=boolean  RndMeth=Simplest
  Relational Operator2 : RelationalOperator  Operator===  OutDataTypeStr=boolean  RndMeth=Simplest
  SRSReq1 : MSMLib/SRSReq  SystemSampleTime=-1
  SRSReq2 : MSMLib/SRSReq  SystemSampleTime=-1
  Switch{,1..3} (4 alike) : Switch  Criteria=u2 > Threshold
  Unit Delay1 : UnitDelay  InitialCondition=g  SampleTime=-1
  Unit Delay{2..4,6,9..10} (6 alike) : UnitDelay  SampleTime=-1
  Unit Delay11 : UnitDelay  InitialCondition=d  SampleTime=-1
  Unit Delay17 : UnitDelay  InitialCondition=d  SampleTime=-1
  Unit Delay5 : UnitDelay  InitialCondition=e  SampleTime=-1
  Unit Delay7 : UnitDelay  InitialCondition=g  SampleTime=-1
  Unit Delay8 : UnitDelay  InitialCondition=e  SampleTime=-1
  SRSLgrstOpenRtIntCnt : Outport
  SRSLgrstCloseRtIntCnt : Outport  Port=2
  LgrstOpenRtMdReq : Outport  Port=3
  LgrstOpenRtSoftInt : Outport  Port=4
  LgrstOpenRtSrcReqTp : Outport  Port=5
  LgrstCloseRtMdReq : Outport  Port=6
  LgrstCloseRtSoftInt : Outport  Port=7
  LgrstCloseRtSrcReqTp : Outport  Port=8
  Notf1ChimeEventStat : Outport  Port=9
  wires:
  Constant12/1 -> Equal1/2, Equal2/2
  Equal2/1 -> AND4/2
  Equal4/1 -> AND3/1
  SRSActiveValidTm/1 -> [SRSActiveValidTm]
  curMode/1 -> [curMode]
  Equal1/1 -> AND4/1
  Constant15/1 -> Equal4/2, Equal5/2
  Unit Delay4/1 -> Equal5/1
  SRSSlctSwReq/1 -> [SRSSlctSwReq]
  PassLgrstOpenRtMdReq/1 -> Unit Delay4/1, Equal4/1
  SRSMode/1 -> [SRSMode]
  AND4/1 -> [PassLgrstCloseRtMdReq]
  AND3/1 -> [PassLgrstOpenRtMdReq]
  PassCmprtMdHMIReqExt/1 -> [PassCmprtMdHMIReqExt]
  Equal5/1 -> AND3/2
  PassLgrstCloseRtMdReq/1 -> Unit Delay6/1, Equal1/1
  Unit Delay6/1 -> Equal2/1
  SRSCnfmSwReq/1 -> [SRSCnfmSwReq]
  Relational Operator1/1 -> AND5/1
  Constant2/1 -> Relational Operator1/2
  Constant6/1 -> Equal9/2
  Unit Delay7/1 -> Equal9/1
  AND5/1 -> [passCmprtMdHMIReq_LgrstOpenRt]
  [PassCmprtMdHMIReqExt] -> Unit Delay7/1, Relational Operator1/1
  Equal9/1 -> AND5/2
  [PassCmprtMdHMIReqExt] -> Unit Delay1/1, Relational Operator2/1
  Equal3/1 -> AND1/2
  Constant3/1 -> Equal3/2
  Unit Delay1/1 -> Equal3/1
  AND1/1 -> [passCmprtMdHMIReq_LgrstCloseRt]
  Constant1/1 -> Relational Operator2/2
  Relational Operator2/1 -> AND1/1
  ButtonLongPressed2/2(mdInterruptCnt) -> SRSLgrstCloseRtIntCnt/1
  [SRSMode] -> Unit Delay17/1
  Unit Delay17/1 -> ButtonLongPressed4/6(SRSMode)
  Constant16/1 -> ButtonLongPressed4/4(CmpReq), SRSReq2/4
  [SRSActiveValidTm] -> SRSReq2/2
  ButtonLongPressed4/1(mdReq) -> [SRSLgrstOpenRtReq]
  [SRSCnfmSwReq] -> ButtonLongPressed4/5(SRSCnfmSwReq), SRSReq2/3
  [curMode] -> ButtonLongPressed2/3(curMdState)
  [SRSSlctSwReq] -> SRSReq2/1
  [curMode] -> ButtonLongPressed4/3(curMdState)
  Constant17/1 -> ButtonLongPressed4/2(longPressThrshhldTm)
  SRSReq2/1 -> ButtonLongPressed4/1(modeReq)
  [SRSCnfmSwReq] -> ButtonLongPressed2/5(SRSCnfmSwReq), SRSReq1/3
  Constant5/1 -> ButtonLongPressed2/2(longPressThrshhldTm)
  [SRSSlctSwReq] -> SRSReq1/1
  [SRSActiveValidTm] -> SRSReq1/2
  ButtonLongPressed2/1(mdReq) -> [SRSLgrstCloseRtReq]
  [SRSMode] -> Unit Delay11/1
  Constant4/1 -> ButtonLongPressed2/4(CmpReq), SRSReq1/4
  SRSReq1/1 -> ButtonLongPressed2/1(modeReq)
  ButtonLongPressed4/2(mdInterruptCnt) -> SRSLgrstOpenRtIntCnt/1
  Unit Delay11/1 -> ButtonLongPressed2/6(SRSMode)
  [passCmprtMdHMIReq_LgrstOpenRt] -> ConfirmRequireSource/4, OR2/3, OR1/3
  Ground2/1 -> ConfirmRequireSource1/2, ConfirmRequireSource1/1
  NOT/1 -> AND2/2
  Switch2/1 -> LgrstCloseRtMdReq/1, Unit Delay9/1
  [HMI2RReq_LgrstOpenRt] -> ConfirmRequireSource/3, OR2/2, OR1/2
  [PassLgrstCloseRtMdReq] -> ConfirmRequireSource1/5, OR4/1, OR3/1
  OR2/1 -> Switch1/1
  [LgrstOpenRtNotf1ChimeEventStat] -> OR/1
  OR/1 -> Notf1ChimeEventStat/1
  ConfirmRequireSource1/1 -> LgrstCloseRtSrcReqTp/1
  [HMI2RReq_LgrstCloseRt] -> ConfirmRequireSource1/3, OR4/2, OR3/2
  LgrstCloseRtMdAvl/1 -> Switch3/2, NOT1/1, Switch2/2
  OR3/1 -> AND7/1, Switch2/1
  OR4/1 -> Switch3/1
  OR1/1 -> AND2/1, Switch/1
  [PassLgrstOpenRtMdReq] -> ConfirmRequireSource/5, OR2/1, OR1/1
  Switch1/1 -> LgrstOpenRtSoftInt/1, Unit Delay3/1
  Switch3/1 -> LgrstCloseRtSoftInt/1, Unit Delay10/1
  LgrstOpenRtMdAvl/1 -> Switch1/2, NOT/1, Switch/2
  [SRSLgrstCloseRtReq] -> ConfirmRequireSource1/6, OR3/4
  Unit Delay10/1 -> Switch3/3
  Unit Delay9/1 -> Switch2/3
  Unit Delay2/1 -> Switch/3
  [LgrstCloseRtNotf1ChimeEventStat] -> OR/2
  AND2/1 -> [LgrstOpenRtNotf1ChimeEventStat]
  AND7/1 -> [LgrstCloseRtNotf1ChimeEventStat]
  [SRSLgrstOpenRtReq] -> ConfirmRequireSource/6, OR1/4
  Ground1/1 -> ConfirmRequireSource/2, ConfirmRequireSource/1
  Switch/1 -> LgrstOpenRtMdReq/1, Unit Delay2/1
  NOT1/1 -> AND7/2
  Unit Delay3/1 -> Switch1/3
  [passCmprtMdHMIReq_LgrstCloseRt] -> ConfirmRequireSource1/4, OR4/3, OR3/3
  ConfirmRequireSource/1 -> LgrstOpenRtSrcReqTp/1
  Constant14/1 -> Equal8/2, Equal7/2
  LgrstOpenRtMdHMI2RRclReq/1 -> Unit Delay5/1, Equal/1
  Unit Delay5/1 -> Equal6/1
  Equal6/1 -> AND/2
  AND6/1 -> [HMI2RReq_LgrstCloseRt]
  Unit Delay8/1 -> Equal8/1
  Equal8/1 -> AND6/2
  AND/1 -> [HMI2RReq_LgrstOpenRt]
  Equal7/1 -> AND6/1
  Equal/1 -> AND/1
  Constant7/1 -> Equal6/2, Equal/2
  LgrstCloseRtMdHMI2RRclReq/1 -> Unit Delay8/1, Equal7/1

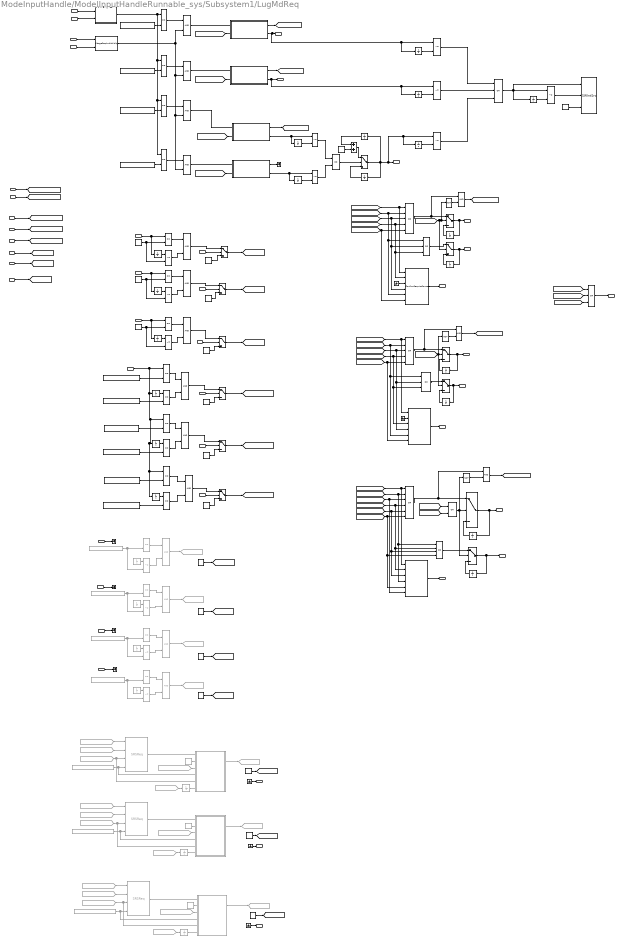
== system ModeInputHandle/ModelInputHandleRunnable_sys/Subsystem1/LugMdReq ==
  note: // PassAcsMdExt ---》 remote
  SlctSwReq : Inport
  SlctSwReqV : Inport  Port=2
  SwConfmReq : Inport  Port=3
  SwConfmReqV : Inport  Port=4
  PassLugMdLtReq : Inport  Port=5
  PassLugMdRtReq : Inport  Port=6
  PassLugAllReq : Inport  Port=7
  passCmprtMdHMIReq : Inport  Port=8
  SRSSlctSwReq : Inport  Port=9
  SRSCnfmSwReq : Inport  Port=10
  SRSActiveValidTm : Inport  Port=11
  buttonLongPressedThrshhldTm : Inport  Port=12
  curMode : Inport  Port=13
  LugMdLtAvl : Inport  Port=14
  LugMdRtAvl : Inport  Port=15
  SRSMode : Inport  Port=16
  HMI2LRclReq : Inport  Port=17
  HMI2RRclReq : Inport  Port=18
  LugAll2LHMIRclReq : Inport  Port=19
  LugAll2RHMIRclReq : Inport  Port=20
  StPassCmprtMdCtrl_Md3_VCUConfig : Inport  Port=21
  StPassCmprtMdCtrl_Md8_VCUConfig : Inport  Port=22
  StPassCmprtMdCtrl_Md9_VCUConfig : Inport  Port=23
  StSrv_StMd3_Config : Inport  Port=24
  StSrv_StMd8_Config : Inport  Port=25
  StSrv_StMd9_Config : Inport  Port=26
  AND{,1..7,9..12,17} (13 alike) : Logic  AllPortsSameDT=off  OutDataTypeStr=boolean
  AND{13..16} (4 alike) : Logic  Commented=on  AllPortsSameDT=off  OutDataTypeStr=boolean
  AND8 : Logic  Operator=OR  AllPortsSameDT=off  OutDataTypeStr=boolean
  Add : Sum
  ButtonLongPressed : Subsystem  AncestorBlock=MSMLib/ButtonLongPressed
  ButtonLongPressed1 : Subsystem  AncestorBlock=MSMLib/ButtonLongPressed
  ButtonLongPressed2 : Subsystem  AncestorBlock=MSMLib/ButtonLongPressed
  ButtonLongPressed3 : Subsystem  Commented=on  AncestorBlock=MSMLib/ButtonLongPressed
  ButtonLongPressed4 : Subsystem  Commented=on  AncestorBlock=MSMLib/ButtonLongPressed
  ButtonLongPressed5 : Subsystem  Commented=on  AncestorBlock=MSMLib/ButtonLongPressed
  ButtonLongPressed6 : Subsystem  AncestorBlock=MSMLib/ButtonLongPressed
  ConfirmRequireSource : MSMLib/ConfirmRequireSource  SystemSampleTime=-1
  ConfirmRequireSource1 : MSMLib/ConfirmRequireSource  SystemSampleTime=-1
  ConfirmRequireSource2 : MSMLib/ConfirmRequireSource  SystemSampleTime=-1
  Constant : Constant  Value=LugSelectSw1.LugSelectSw_Left  OutDataTypeStr=Enum: LugSelectSw1
  Constant1 : Constant  Value=LugSelectSw1.LugSelectSw_Right  OutDataTypeStr=Enum: LugSelectSw1
  Constant10 : Constant  Commented=on  Value=SRSMode1.SRSSlctSwStat_LfLug  OutDataTypeStr=Enum:SRSMode1
  Constant11 : Constant  Commented=on  Value=0  OutDataTypeStr=uint8
  Constant12 : Constant  Commented=on  Value=SRSMode1.SRSSlctSwStat_AllLug  OutDataTypeStr=Enum:SRSMode1
  Constant13 : Constant  Commented=on  Value=0  OutDataTypeStr=uint8
  Constant14 : Constant  Value=CmprtMdHMIReqTp1.CmprtMdHMIReqTp_NoAction  OutDataTypeStr=Enum:CmprtMdHMIReqTp1
  Constant15 : Constant  Value=CmprtMdHMIReqTp1.CmprtMdHMIReqTp_NoAction  OutDataTypeStr=Enum:CmprtMdHMIReqTp1
  Constant{16..19} (4 alike) : Constant  Commented=on  Value=MdReqTp1.MdReqTp_Start
  Constant2 : Constant  Value=LugSelectSw1.LugSelectSw_All  OutDataTypeStr=Enum: LugSelectSw1
  Constant20 : Constant  Value=true  OutDataTypeStr=boolean
  Constant21 : Constant  Value=CmprtMdHMIReqTp1.CmprtMdHMIReqTp_NoAction  OutDataTypeStr=Enum:CmprtMdHMIReqTp1
  Constant22 : Constant  Value=LugSelectSw1.LugSelectSw_NoAction  OutDataTypeStr=Enum: LugSelectSw1
  Constant23 : Constant  OutDataTypeStr=uint8
  Constant24 : Constant  Value=4  OutDataTypeStr=uint8
  Constant{25..37} (13 alike) : Constant  Value=0  OutDataTypeStr=boolean
  Constant3 : Constant  Value=true  OutDataTypeStr=boolean
  Constant4 : Constant  Value=true  OutDataTypeStr=boolean
  Constant5 : Constant  Value=CmprtMdHMIReqTp1.CmprtMdHMIReqTp_Mode8  OutDataTypeStr=Enum:CmprtMdHMIReqTp1
  Constant6 : Constant  Value=CmprtMdHMIReqTp1.CmprtMdHMIReqTp_Mode9  OutDataTypeStr=Enum:CmprtMdHMIReqTp1
  Constant7 : Constant  Value=CmprtMdHMIReqTp1.CmprtMdHMIReqTp_Mode3  OutDataTypeStr=Enum:CmprtMdHMIReqTp1
  Constant8 : Constant  Commented=on  Value=SRSMode1.SRSSlctSwStat_RtLug  OutDataTypeStr=Enum:SRSMode1
  Constant9 : Constant  Commented=on  Value=0  OutDataTypeStr=uint8
  Equal{,1,3..4,6..8,17} (8 alike) : RelationalOperator  Operator===  OutDataTypeStr=boolean  RndMeth=Simplest
  Equal{10,12,14,16} (4 alike) : RelationalOperator  Commented=on  Operator=~=  OutDataTypeStr=boolean  RndMeth=Simplest
  Equal{9,11,13,15} (4 alike) : RelationalOperator  Commented=on  Operator===  OutDataTypeStr=boolean  RndMeth=Simplest
  Equal{2,5,18..24} (9 alike) : RelationalOperator  Operator=~=  OutDataTypeStr=boolean  RndMeth=Simplest
  From10 : From  Commented=on  GotoTag=curMode
  From11 : From  Commented=on  GotoTag=SRSSlctSwReq
  From12 : From  Commented=on  GotoTag=SRSActiveValidTm
  From13 : From  Commented=on  GotoTag=SRSSlctSwReq
  From14 : From  Commented=on  GotoTag=SRSActiveValidTm
  From15 : From  Commented=on  GotoTag=SRSCnfmSwReq
  From16 : From  Commented=on  GotoTag=SRSCnfmSwReq
  From17 : From  Commented=on  GotoTag=curMode
  From42 : From  Commented=on  GotoTag=SRSMode
  From43 : From  Commented=on  GotoTag=SRSMode
  From44 : From  Commented=on  GotoTag=SRSMode
  From6 : From  Commented=on  GotoTag=curMode
  From7 : From  Commented=on  GotoTag=SRSSlctSwReq
  From8 : From  Commented=on  GotoTag=SRSActiveValidTm
  From9 : From  Commented=on  GotoTag=SRSCnfmSwReq
  Goto11 : Goto  Commented=on  GotoTag=SRSLfLugReq
  Goto15 : Goto  Commented=on  GotoTag=SRSRtLugReq
  Goto17 : Goto  Commented=on  GotoTag=SRSAllLugReq
  Goto21 : Goto  Commented=on  GotoTag=HMI2RReq
  Goto22 : Goto  Commented=on  GotoTag=HMI2LReq
  Goto23 : Goto  Commented=on  GotoTag=LugAllHMI2LReq
  Goto24 : Goto  Commented=on  GotoTag=LugAllHMI2RReq
  Ground{,1..4} (5 alike) : Ground
  NOT : Logic  Operator=NOT  AllPortsSameDT=off  OutDataTypeStr=boolean
  NOT1 : Logic  Operator=NOT  AllPortsSameDT=off  OutDataTypeStr=boolean
  NOT2 : Logic  Operator=NOT  AllPortsSameDT=off  OutDataTypeStr=boolean
  OR : Logic  Operator=OR  Inputs=5  AllPortsSameDT=off  OutDataTypeStr=boolean
  OR1 : Logic  Operator=OR  Inputs=5  AllPortsSameDT=off  OutDataTypeStr=boolean
  OR2 : Logic  Operator=OR  Inputs=6  AllPortsSameDT=off  OutDataTypeStr=boolean
  OR{3..5,8} (4 alike) : Logic  Operator=OR  Inputs=3  AllPortsSameDT=off  OutDataTypeStr=boolean
  OR6 : Logic  Operator=OR  AllPortsSameDT=off  OutDataTypeStr=boolean
  OR7 : Logic  Operator=OR  Inputs=4  AllPortsSameDT=off  OutDataTypeStr=boolean
  Relational Operator{,1..4} (5 alike) : RelationalOperator  Operator===  OutDataTypeStr=boolean  RndMeth=Simplest
  SRSReq1 : MSMLib/SRSReq  Commented=on  SystemSampleTime=-1
  SRSReq2 : MSMLib/SRSReq  Commented=on  SystemSampleTime=-1
  SRSReq3 : MSMLib/SRSReq  Commented=on  SystemSampleTime=-1
  SWIntSrc : MSMLib/SWIntSrc  SystemSampleTime=-1
  Subsystem1 : Subsystem
  Subsystem2 : MSMLib/MergeReqAndValidity  SystemSampleTime=-1
  Switch{,1..12} (13 alike) : Switch  Criteria=u2 > Threshold
  Terminator_{1..4,44} (5 alike) : Terminator
  Unit Delay : UnitDelay  InitialCondition=c  SampleTime=-1
  Unit Delay{1..2,5..10,16,19..26} (17 alike) : UnitDelay  SampleTime=-1
  Unit Delay11 : UnitDelay  Commented=on  InitialCondition=d  SampleTime=-1
  Unit Delay{12..15} (4 alike) : UnitDelay  Commented=on  InitialCondition=e  SampleTime=-1
  Unit Delay17 : UnitDelay  Commented=on  InitialCondition=d  SampleTime=-1
  Unit Delay18 : UnitDelay  Commented=on  InitialCondition=d  SampleTime=-1
  Unit Delay3 : UnitDelay  InitialCondition=c  SampleTime=-1
  Unit Delay4 : UnitDelay  InitialCondition=c  SampleTime=-1
  LtLugMdReq : Outport
  RtLugMdReq : Outport  Port=2
  AllLugMdReq : Outport  Port=3
  LtLugSrcReqTp : Outport  Port=4
  RtLugSrcReqTp : Outport  Port=5
  AllLugSrcReqTp : Outport  Port=6
  SwLtLugIntCnt : Outport  Port=7
  SwRtLugIntCnt : Outport  Port=8
  SwAllLugIntCnt : Outport  Port=9
  SRSAllLugIntCnt : Outport  Port=10
  Notf1ChimeEventStat : Outport  Port=11
  LtLugSoftInt : Outport  Port=12
  RtLugSoftInt : Outport  Port=13
  AllLugSoftInt : Outport  Port=14
  SRSLfLugIntCnt : Outport  Port=15
  SRSRtLugIntCnt : Outport  Port=16
  wires:
  SRSSlctSwReq/1 -> [SRSSlctSwReq]
  buttonLongPressedThrshhldTm/1 -> [buttonLongPressedThrshhldTm]
  SRSCnfmSwReq/1 -> [SRSCnfmSwReq]
  SRSActiveValidTm/1 -> [SRSActiveValidTm]
  curMode/1 -> [curMode]
  SlctSwReq/1 -> Subsystem1/1(src)
  SlctSwReqV/1 -> Subsystem1/2(vadility)
  Constant/1 -> Relational Operator/2
  [buttonLongPressedThrshhldTm] -> ButtonLongPressed/2(longPressThrshhldTm)
  ButtonLongPressed/1(mdReq) -> [SwLtLugReq]
  SwConfmReq/1 -> Subsystem2/1
  SwConfmReqV/1 -> Subsystem2/2
  Subsystem2/1 -> AND12/2, AND2/2, AND1/2, AND/2
  Relational Operator/1 -> AND/1
  AND/1 -> ButtonLongPressed/1(modeReq)
  Constant1/1 -> Relational Operator1/2
  Relational Operator1/1 -> AND1/1
  AND1/1 -> ButtonLongPressed1/1(modeReq)
  [buttonLongPressedThrshhldTm] -> ButtonLongPressed1/2(longPressThrshhldTm)
  ButtonLongPressed1/1(mdReq) -> [SwRtLugReq]
  Constant2/1 -> Relational Operator2/2
  Relational Operator2/1 -> AND2/1
  [buttonLongPressedThrshhldTm] -> ButtonLongPressed2/2(longPressThrshhldTm)
  ButtonLongPressed2/1(mdReq) -> [SwAllLugReq]
  Equal4/1 -> AND3/1
  Constant4/1 -> Equal4/2, Equal5/2
  Equal5/1 -> AND3/2
  PassLugMdLtReq/1 -> Unit Delay2/1, Equal4/1
  Unit Delay2/1 -> Equal5/1
  Equal2/1 -> AND4/2
  Constant3/1 -> Equal1/2, Equal2/2
  PassLugMdRtReq/1 -> Unit Delay1/1, Equal1/1
  Equal1/1 -> AND4/1
  Unit Delay1/1 -> Equal2/1
  Relational Operator3/1 -> AND5/1
  Equal6/1 -> AND5/2
  Unit Delay3/1 -> Equal6/1
  Constant5/1 -> Relational Operator3/2
  passCmprtMdHMIReq/1 -> Unit Delay4/1, Equal7/1, Unit Delay/1, Equal/1, Unit Delay3/1, Relational Operator3/1
  Constant6/1 -> Equal/2
  Unit Delay/1 -> Equal3/1
  Equal/1 -> AND6/1
  Equal3/1 -> AND6/2
  Constant7/1 -> Equal7/2
  Unit Delay4/1 -> Equal8/1
  Equal7/1 -> AND7/1
  Equal8/1 -> AND7/2
  From15/1 -> ButtonLongPressed4/5(SRSCnfmSwReq), SRSReq2/3
  Constant9/1 -> ButtonLongPressed4/2(longPressThrshhldTm)
  Constant8/1 -> ButtonLongPressed4/4(CmpReq), SRSReq2/4
  From13/1 -> SRSReq2/1
  From14/1 -> SRSReq2/2
  ButtonLongPressed4/1(mdReq) -> Goto15/1
  SRSReq2/1 -> ButtonLongPressed4/1(modeReq)
  From6/1 -> ButtonLongPressed4/3(curMdState)
  From7/1 -> SRSReq1/1
  SRSReq1/1 -> ButtonLongPressed3/1(modeReq)
  Constant11/1 -> ButtonLongPressed3/2(longPressThrshhldTm)
  From9/1 -> ButtonLongPressed3/5(SRSCnfmSwReq), SRSReq1/3
  Constant10/1 -> ButtonLongPressed3/4(CmpReq), SRSReq1/4
  From8/1 -> SRSReq1/2
  From10/1 -> ButtonLongPressed3/3(curMdState)
  ButtonLongPressed3/1(mdReq) -> Goto11/1
  From11/1 -> SRSReq3/1
  SRSReq3/1 -> ButtonLongPressed5/1(modeReq)
  Constant13/1 -> ButtonLongPressed5/2(longPressThrshhldTm)
  Constant12/1 -> ButtonLongPressed5/4(CmpReq), SRSReq3/4
  From12/1 -> SRSReq3/2
  From17/1 -> ButtonLongPressed5/3(curMdState)
  ButtonLongPressed5/1(mdReq) -> Goto17/1
  From16/1 -> ButtonLongPressed5/5(SRSCnfmSwReq), SRSReq3/3
  [SwLtLugReq] -> OR/1, ConfirmRequireSource/1
  [PassLugMdLtReq] -> OR/2, ConfirmRequireSource/5, OR4/1
  [passCmprtMdHMIReq_LtLug] -> OR/3, ConfirmRequireSource/4, OR4/2
  OR/1 -> Switch/1, AND9/1
  Switch/1 -> Unit Delay5/1, LtLugMdReq/1
  Unit Delay5/1 -> Switch/3
  ConfirmRequireSource/1 -> LtLugSrcReqTp/1
  [SwRtLugReq] -> OR1/1, ConfirmRequireSource1/1
  [PassLugMdRtReq] -> OR1/2, ConfirmRequireSource1/5, OR5/1
  [passCmprtMdHMIReq_RtLug] -> ConfirmRequireSource1/4, OR5/2, OR1/3
  OR1/1 -> AND10/1, Switch1/1
  Switch1/1 -> Unit Delay6/1, RtLugMdReq/1
  Unit Delay6/1 -> Switch1/3
  ConfirmRequireSource1/1 -> RtLugSrcReqTp/1
  [SwAllLugReq] -> ConfirmRequireSource2/1, OR2/1
  [SRSAllLugReq] -> ConfirmRequireSource2/6, OR2/3
  OR2/1 -> AND11/1, Switch2/1
  LugMdLtAvl/1 -> [LugMdLtAvl]
  LugMdRtAvl/1 -> [LugMdRtAvl]
  [LugMdLtAvl] -> Switch3/2, Switch/2, NOT/1
  [LugMdRtAvl] -> NOT1/1, Switch1/2, Switch4/2
  [LugMdLtAvl] -> AND8/1
  [LugMdRtAvl] -> AND8/2
  AND8/1 -> NOT2/1, Switch5/2, Switch2/2
  Switch2/1 -> Unit Delay7/1, AllLugMdReq/1
  Unit Delay7/1 -> Switch2/3
  ConfirmRequireSource2/1 -> AllLugSrcReqTp/1
  NOT/1 -> AND9/2
  AND9/1 -> [LtLugMdNotf1ChimeEventStat]
  NOT1/1 -> AND10/2
  AND10/1 -> [RtLugMdNotf1ChimeEventStat]
  [LtLugMdNotf1ChimeEventStat] -> OR3/1
  [RtLugMdNotf1ChimeEventStat] -> OR3/2
  OR3/1 -> Notf1ChimeEventStat/1
  OR4/1 -> Switch3/1
  Unit Delay8/1 -> Switch3/3
  Switch3/1 -> Unit Delay8/1, LtLugSoftInt/1
  Switch4/1 -> Unit Delay9/1, RtLugSoftInt/1
  OR5/1 -> Switch4/1
  Unit Delay9/1 -> Switch4/3
  Switch5/1 -> Unit Delay10/1, AllLugSoftInt/1
  Unit Delay10/1 -> Switch5/3
  [passCmprtMdHMIReq_AllLug] -> OR7/1, ConfirmRequireSource2/4, OR2/2
  Unit Delay11/1 -> ButtonLongPressed5/6(SRSMode)
  [AllLugMdNotf1ChimeEventStat] -> OR3/3
  Ground/1 -> ConfirmRequireSource/3
  Ground1/1 -> ConfirmRequireSource1/2
  Unit Delay12/1 -> Equal10/1
  Equal10/1 -> AND13/2
  Equal11/1 -> AND14/1
  Equal9/1 -> AND13/1
  Constant17/1 -> Equal12/2, Equal11/2
  AND13/1 -> Goto22/1
  AND14/1 -> Goto21/1
  Unit Delay13/1 -> Equal12/1
  Equal12/1 -> AND14/2
  Constant16/1 -> Equal10/2, Equal9/2
  Equal14/1 -> AND15/2
  Constant18/1 -> Equal14/2, Equal13/2
  AND15/1 -> Goto23/1
  Unit Delay14/1 -> Equal14/1
  Equal13/1 -> AND15/1
  AND16/1 -> Goto24/1
  Equal16/1 -> AND16/2
  Equal15/1 -> AND16/1
  Unit Delay15/1 -> Equal16/1
  Constant19/1 -> Equal16/2, Equal15/2
  [HMI2LReq] -> ConfirmRequireSource/2, OR4/3, OR/4
  [HMI2RReq] -> OR1/4, OR5/3, ConfirmRequireSource1/3
  [LugAllHMI2LReq] -> OR7/2, ConfirmRequireSource2/2, OR2/4
  [LugAllHMI2RReq] -> ConfirmRequireSource2/3, OR7/3, OR2/5
  OR7/1 -> Switch5/1
  Equal18/1 -> AND17/2
  Equal17/1 -> AND17/1
  Constant20/1 -> Equal17/2, Equal18/2
  PassLugAllReq/1 -> Unit Delay16/1, Equal17/1
  Unit Delay16/1 -> Equal18/1
  [PassLugAllReq] -> OR7/4, ConfirmRequireSource2/5, OR2/6
  [SRSLfLugReq] -> ConfirmRequireSource/6, OR/5
  [SRSRtLugReq] -> ConfirmRequireSource1/6, OR1/5
  SRSMode/1 -> [SRSMode]
  From42/1 -> Unit Delay11/1
  From43/1 -> Unit Delay17/1
  Unit Delay17/1 -> ButtonLongPressed4/6(SRSMode)
  From44/1 -> Unit Delay18/1
  Unit Delay18/1 -> ButtonLongPressed3/6(SRSMode)
  Constant14/1 -> Equal6/2
  Constant15/1 -> Equal3/2
  Constant21/1 -> Equal8/2
  NOT2/1 -> AND11/2
  AND11/1 -> [AllLugMdNotf1ChimeEventStat]
  Subsystem1/1(req) -> Relational Operator4/1, Relational Operator2/1, Relational Operator1/1, Relational Operator/1
  Constant22/1 -> Relational Operator4/2
  Relational Operator4/1 -> AND12/1
  ButtonLongPressed/2(mdInterruptCnt) -> Unit Delay23/1, Equal21/1, SwLtLugIntCnt/1
  ButtonLongPressed1/2(mdInterruptCnt) -> Unit Delay24/1, Equal22/1, SwRtLugIntCnt/1
  AND2/1 -> ButtonLongPressed2/1(modeReq)
  AND12/1 -> ButtonLongPressed6/1(modeReq)
  [buttonLongPressedThrshhldTm] -> ButtonLongPressed6/2(longPressThrshhldTm)
  ButtonLongPressed6/1(mdReq) -> Terminator_44/1
  ButtonLongPressed2/2(mdInterruptCnt) -> Unit Delay19/1, Equal19/1
  Unit Delay19/1 -> Equal19/2
  Unit Delay20/1 -> Equal20/2
  ButtonLongPressed6/2(mdInterruptCnt) -> Unit Delay20/1, Equal20/1
  Equal19/1 -> OR6/1
  Equal20/1 -> OR6/2
  Constant23/1 -> Add/2
  OR6/1 -> Switch6/2
  Switch6/1 -> Unit Delay22/1, Unit Delay21/1, Unit Delay25/1, Equal23/1, SwAllLugIntCnt/1
  Add/1 -> Switch6/1
  Unit Delay21/1 -> Switch6/3
  Unit Delay22/1 -> Add/1
  Unit Delay23/1 -> Equal21/2
  Unit Delay24/1 -> Equal22/2
  Unit Delay25/1 -> Equal23/2
  Equal22/1 -> OR8/2
  Equal21/1 -> OR8/1
  Equal23/1 -> OR8/3
  OR8/1 -> SWIntSrc/1, Unit Delay26/1, Equal24/1
  Unit Delay26/1 -> Equal24/2
  Equal24/1 -> SWIntSrc/2
  Constant24/1 -> SWIntSrc/3
  HMI2LRclReq/1 -> Terminator_3/1
  HMI2RRclReq/1 -> Terminator_1/1
  LugAll2LHMIRclReq/1 -> Terminator_2/1
  LugAll2RHMIRclReq/1 -> Terminator_4/1
  Ground2/1 -> SRSLfLugIntCnt/1
  Ground3/1 -> SRSRtLugIntCnt/1
  Ground4/1 -> SRSAllLugIntCnt/1
  Constant25/1 -> [HMI2LReq]
  Constant26/1 -> [HMI2RReq]
  Constant27/1 -> [LugAllHMI2LReq]
  Constant28/1 -> [LugAllHMI2RReq]
  Constant29/1 -> [SRSLfLugReq]
  Constant30/1 -> [SRSRtLugReq]
  Constant31/1 -> [SRSAllLugReq]
  StSrv_StMd8_Config/1 -> Switch7/2
  AND3/1 -> Switch7/1
  Constant32/1 -> Switch7/3
  Switch7/1 -> [PassLugMdLtReq]
  StSrv_StMd9_Config/1 -> Switch8/2
  Constant33/1 -> Switch8/3
  AND4/1 -> Switch8/1
  Switch8/1 -> [PassLugMdRtReq]
  StSrv_StMd3_Config/1 -> Switch9/2
  AND17/1 -> Switch9/1
  Constant34/1 -> Switch9/3
  Switch9/1 -> [PassLugAllReq]
  StPassCmprtMdCtrl_Md8_VCUConfig/1 -> Switch10/2
  AND5/1 -> Switch10/1
  Constant35/1 -> Switch10/3
  Switch10/1 -> [passCmprtMdHMIReq_LtLug]
  StPassCmprtMdCtrl_Md9_VCUConfig/1 -> Switch11/2
  AND6/1 -> Switch11/1
  Switch11/1 -> [passCmprtMdHMIReq_RtLug]
  Constant36/1 -> Switch11/3
  StPassCmprtMdCtrl_Md3_VCUConfig/1 -> Switch12/2
  AND7/1 -> Switch12/1
  Constant37/1 -> Switch12/3
  Switch12/1 -> [passCmprtMdHMIReq_AllLug]
